simulink model "model2"  (R2024b)
settings: Solver=VariableStepAuto  StartTime=0.0  StopTime=10  RelTol=1e-3
InitFcn:
  | run("init.m")
values from neighbouring files (symbols this model uses):
  A = 1 / (C1 + (C2 * g / C4))    (= 0.0106647300931)    [init.m]    (also in state_var_model_kean.m = [0, 1, 0, 0)
  B = (C2 * g) / (C4 * C1 + C2 * g)    (= 0.0749412852736)    [init.m]    (also in state_var_model_kean.m = [0, 0)
  beta = 0.2    [init.m]
  C = C2 / (C4 * C1 + C2^2)    (= 0.0058277612604)    [init.m]
  D = (C2 * g) / (C4 + (C2^2 / C1))    (= 4.95895525682)    [init.m]
  Ft = 170    [init.m]
settings Model: Creator=sengu  LastModifiedBy=sengu

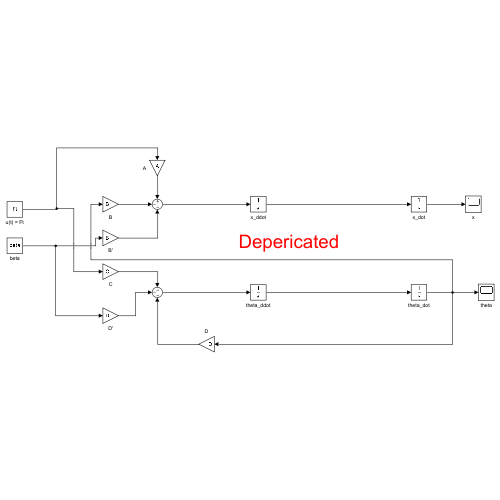
[thumbnail: Simulink's stored preview of the top-level diagram]
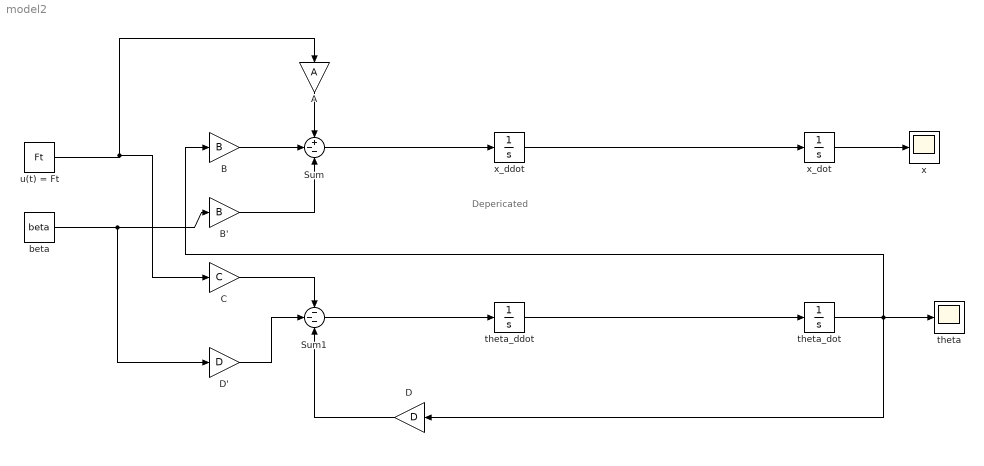
== system model2 ==
  note: Depericated
  A : Gain  Gain=A
  B : Gain  Gain=B
  B' : Gain  Gain=B
  C : Gain  Gain=C
  D : Gain  Gain=D
  D' : Gain  Gain=D
  Sum : Sum  Inputs=+--
  Sum1 : Sum  Inputs=---
  beta : Constant  Value=beta
  theta : Scope
  theta_ddot : Integrator
  theta_dot : Integrator
  u(t) = Ft : Constant  Value=Ft
  x : Scope
  x_ddot : Integrator
  x_dot : Integrator
  wires:
  Sum/1 -> x_ddot/1
  x_ddot/1 -> x_dot/1
  theta_ddot/1 -> theta_dot/1
  theta_dot/1 -> D/1, B/1, theta/1
  x_dot/1 -> x/1
  u(t) = Ft/1 -> C/1, A/1
  A/1 -> Sum/1
  B/1 -> Sum/2
  beta/1 -> D'/1, B'/1
  B'/1 -> Sum/3
  C/1 -> Sum1/1
  D/1 -> Sum1/3
  D'/1 -> Sum1/2
  Sum1/1 -> theta_ddot/1
